simulink model "Two_Zone_MVDC_PSolver"  (R2025b)
settings: Solver=FixedStepDiscrete  StartTime=0.0  StopTime=30  FixedStep=TsELEC  RelTol=1e-3  EnableMultiTasking=on
InitFcn:
  | TsELEC = 25e-6;
  | Ts = 25e-6;
undefined symbols (not defined in the file or in its folder): DiscIntNeverNeededParam, ee_sli_rtmsupport, GABDA, GABDB, GBBDA, GBBDB, gcbh, GPPMA, GPPMB, GPPMC, SADA, SADB, SADC, SADD, SBDA, SBDB, SBDC, SCDA, SCDB, SCDC, SCDD, SDDA, SDDB, SDDC, SDDD, SDDE, TsCont
libraries: fl_lib x97, nesl_utility x73, ee_lib x48, simulink x3, slpidlib x3, eeSmAC1C x2, eePowerMeasurement x2, mcbeeMathTransformLib x2, eeTransforms x1
(part 2 of 4)

== system Two_Zone_MVDC_PSolver/SCDC ==
  SADA : ee_lib/Switches & Breakers/DPST Switch  R_closed=1e-4 Ohm  G_open=1e-6 S  Threshold=0.5 V  Width=0 V  model_dynamics=0  t_on=1e-3 s  t_off=1e-3 s  initial_vT=0 V
      settings: InternalSimscapePortConfiguration="{\"Bottom\":[],\"Left\":[{\"id\":\"vT\",\"label\":\"vT\",\"type\":\"input\"},{\"id\":\"p1\",\"label\":\"\",\"type\":\"foundation.electrical.electrical\"},{\"id\":\"p2\",\"label\":\"\",\"type\":\"foundation.electrical.electrical\"}],\"Right\":[{\"id\":\"n1\",\"label\":\"\",\"type\":\"foundation.electrical.electrical\"},{\"id\":\"n2\",\"label\":\"\",\"type\":\"foundation.electrical.electrical\"}],\"Top\":[]}"
  Simulink-PS Converter : nesl_utility/Simulink-PS Converter  PhysicalDomain=network_engine_domain  SubClassName=ps_input  LeftPortType=input  RightPortType=output  PseudoPeriodic=off  Frequencies=[]  NoiseDistribution=none  NoiseParameters=[]  Unit=1  AffineConversion=off  FilteringAndDerivatives=provide  SimscapeFilterOrder=1  InputFilterTimeConstant=0.001  UdotUserProvided=0
  "+ " : PMIOPort  Side=Right
  + : PMIOPort  Port=2  Side=Left
  "- " : PMIOPort  Port=3  Side=Right
  - : PMIOPort  Port=4  Side=Left
  wires:
  [SCDC] -> Simulink-PS Converter/1
  connections:
  SADA/LConn2 -- +/RConn1
  Simulink-PS Converter/RConn1 -- SADA/LConn1
  SADA/RConn2 -- "- "/RConn1
  SADA/LConn3 -- -/RConn1
  SADA/RConn1 -- "+ "/RConn1

== system Two_Zone_MVDC_PSolver/SCDD ==
  SADA : ee_lib/Switches & Breakers/DPST Switch  R_closed=1e-4 Ohm  G_open=1e-6 S  Threshold=0.5 V  Width=0 V  model_dynamics=0  t_on=1e-3 s  t_off=1e-3 s  initial_vT=0 V
      settings: InternalSimscapePortConfiguration="{\"Bottom\":[],\"Left\":[{\"id\":\"vT\",\"label\":\"vT\",\"type\":\"input\"},{\"id\":\"p1\",\"label\":\"\",\"type\":\"foundation.electrical.electrical\"},{\"id\":\"p2\",\"label\":\"\",\"type\":\"foundation.electrical.electrical\"}],\"Right\":[{\"id\":\"n1\",\"label\":\"\",\"type\":\"foundation.electrical.electrical\"},{\"id\":\"n2\",\"label\":\"\",\"type\":\"foundation.electrical.electrical\"}],\"Top\":[]}"
  Simulink-PS Converter : nesl_utility/Simulink-PS Converter  PhysicalDomain=network_engine_domain  SubClassName=ps_input  LeftPortType=input  RightPortType=output  PseudoPeriodic=off  Frequencies=[]  NoiseDistribution=none  NoiseParameters=[]  Unit=1  AffineConversion=off  FilteringAndDerivatives=provide  SimscapeFilterOrder=1  InputFilterTimeConstant=0.001  UdotUserProvided=0
  "+ " : PMIOPort  Side=Right
  + : PMIOPort  Port=2  Side=Left
  "- " : PMIOPort  Port=3  Side=Right
  - : PMIOPort  Port=4  Side=Left
  wires:
  [SCDD] -> Simulink-PS Converter/1
  connections:
  SADA/RConn1 -- "+ "/RConn1
  SADA/LConn3 -- -/RConn1
  SADA/RConn2 -- "- "/RConn1
  Simulink-PS Converter/RConn1 -- SADA/LConn1
  SADA/LConn2 -- +/RConn1

== system Two_Zone_MVDC_PSolver/SDDA ==
  SDDA : ee_lib/Switches & Breakers/DPST Switch  R_closed=1e-4 Ohm  G_open=1e-6 S  Threshold=0.5 V  Width=0 V  model_dynamics=0  t_on=1e-3 s  t_off=1e-3 s  initial_vT=0 V
      settings: InternalSimscapePortConfiguration="{\"Bottom\":[],\"Left\":[{\"id\":\"vT\",\"label\":\"vT\",\"type\":\"input\"},{\"id\":\"p1\",\"label\":\"\",\"type\":\"foundation.electrical.electrical\"},{\"id\":\"p2\",\"label\":\"\",\"type\":\"foundation.electrical.electrical\"}],\"Right\":[{\"id\":\"n1\",\"label\":\"\",\"type\":\"foundation.electrical.electrical\"},{\"id\":\"n2\",\"label\":\"\",\"type\":\"foundation.electrical.electrical\"}],\"Top\":[]}"
  Simulink-PS Converter : nesl_utility/Simulink-PS Converter  PhysicalDomain=network_engine_domain  SubClassName=ps_input  LeftPortType=input  RightPortType=output  PseudoPeriodic=off  Frequencies=[]  NoiseDistribution=none  NoiseParameters=[]  Unit=1  AffineConversion=off  FilteringAndDerivatives=provide  SimscapeFilterOrder=1  InputFilterTimeConstant=0.001  UdotUserProvided=0
  "+ " : PMIOPort  Side=Right
  + : PMIOPort  Port=2  Side=Left
  "- " : PMIOPort  Port=3  Side=Right
  - : PMIOPort  Port=4  Side=Left
  wires:
  [SDDA] -> Simulink-PS Converter/1
  connections:
  SDDA/LConn2 -- +/RConn1
  Simulink-PS Converter/RConn1 -- SDDA/LConn1
  SDDA/RConn2 -- "- "/RConn1
  SDDA/LConn3 -- -/RConn1
  SDDA/RConn1 -- "+ "/RConn1

== system Two_Zone_MVDC_PSolver/SDDB ==
  SDDB : ee_lib/Switches & Breakers/DPST Switch  R_closed=1e-4 Ohm  G_open=1e-6 S  Threshold=0.5 V  Width=0 V  model_dynamics=0  t_on=1e-3 s  t_off=1e-3 s  initial_vT=0 V
      settings: InternalSimscapePortConfiguration="{\"Bottom\":[],\"Left\":[{\"id\":\"vT\",\"label\":\"vT\",\"type\":\"input\"},{\"id\":\"p1\",\"label\":\"\",\"type\":\"foundation.electrical.electrical\"},{\"id\":\"p2\",\"label\":\"\",\"type\":\"foundation.electrical.electrical\"}],\"Right\":[{\"id\":\"n1\",\"label\":\"\",\"type\":\"foundation.electrical.electrical\"},{\"id\":\"n2\",\"label\":\"\",\"type\":\"foundation.electrical.electrical\"}],\"Top\":[]}"
  Simulink-PS Converter : nesl_utility/Simulink-PS Converter  PhysicalDomain=network_engine_domain  SubClassName=ps_input  LeftPortType=input  RightPortType=output  PseudoPeriodic=off  Frequencies=[]  NoiseDistribution=none  NoiseParameters=[]  Unit=1  AffineConversion=off  FilteringAndDerivatives=provide  SimscapeFilterOrder=1  InputFilterTimeConstant=0.001  UdotUserProvided=0
  "+ " : PMIOPort  Side=Right
  + : PMIOPort  Port=2  Side=Left
  "- " : PMIOPort  Port=3  Side=Right
  - : PMIOPort  Port=4  Side=Left
  wires:
  [SDDB] -> Simulink-PS Converter/1
  connections:
  SDDB/RConn1 -- "+ "/RConn1
  SDDB/LConn3 -- -/RConn1
  SDDB/RConn2 -- "- "/RConn1
  Simulink-PS Converter/RConn1 -- SDDB/LConn1
  SDDB/LConn2 -- +/RConn1

== system Two_Zone_MVDC_PSolver/SDDC ==
  SDDC : ee_lib/Switches & Breakers/DPST Switch  R_closed=1e-4 Ohm  G_open=1e-6 S  Threshold=0.5 V  Width=0 V  model_dynamics=0  t_on=1e-3 s  t_off=1e-3 s  initial_vT=0 V
      settings: InternalSimscapePortConfiguration="{\"Bottom\":[],\"Left\":[{\"id\":\"vT\",\"label\":\"vT\",\"type\":\"input\"},{\"id\":\"p1\",\"label\":\"\",\"type\":\"foundation.electrical.electrical\"},{\"id\":\"p2\",\"label\":\"\",\"type\":\"foundation.electrical.electrical\"}],\"Right\":[{\"id\":\"n1\",\"label\":\"\",\"type\":\"foundation.electrical.electrical\"},{\"id\":\"n2\",\"label\":\"\",\"type\":\"foundation.electrical.electrical\"}],\"Top\":[]}"
  Simulink-PS Converter : nesl_utility/Simulink-PS Converter  PhysicalDomain=network_engine_domain  SubClassName=ps_input  LeftPortType=input  RightPortType=output  PseudoPeriodic=off  Frequencies=[]  NoiseDistribution=none  NoiseParameters=[]  Unit=1  AffineConversion=off  FilteringAndDerivatives=provide  SimscapeFilterOrder=1  InputFilterTimeConstant=0.001  UdotUserProvided=0
  "+ " : PMIOPort  Side=Right
  + : PMIOPort  Port=2  Side=Left
  "- " : PMIOPort  Port=3  Side=Right
  - : PMIOPort  Port=4  Side=Left
  wires:
  [SDDC] -> Simulink-PS Converter/1
  connections:
  SDDC/LConn2 -- +/RConn1
  Simulink-PS Converter/RConn1 -- SDDC/LConn1
  SDDC/RConn2 -- "- "/RConn1
  SDDC/LConn3 -- -/RConn1
  SDDC/RConn1 -- "+ "/RConn1

== system Two_Zone_MVDC_PSolver/SDDD ==
  SDDD : ee_lib/Switches & Breakers/DPST Switch  R_closed=1e-4 Ohm  G_open=1e-6 S  Threshold=0.5 V  Width=0 V  model_dynamics=0  t_on=1e-3 s  t_off=1e-3 s  initial_vT=0 V
      settings: InternalSimscapePortConfiguration="{\"Bottom\":[],\"Left\":[{\"id\":\"vT\",\"label\":\"vT\",\"type\":\"input\"},{\"id\":\"p1\",\"label\":\"\",\"type\":\"foundation.electrical.electrical\"},{\"id\":\"p2\",\"label\":\"\",\"type\":\"foundation.electrical.electrical\"}],\"Right\":[{\"id\":\"n1\",\"label\":\"\",\"type\":\"foundation.electrical.electrical\"},{\"id\":\"n2\",\"label\":\"\",\"type\":\"foundation.electrical.electrical\"}],\"Top\":[]}"
  Simulink-PS Converter : nesl_utility/Simulink-PS Converter  PhysicalDomain=network_engine_domain  SubClassName=ps_input  LeftPortType=input  RightPortType=output  PseudoPeriodic=off  Frequencies=[]  NoiseDistribution=none  NoiseParameters=[]  Unit=1  AffineConversion=off  FilteringAndDerivatives=provide  SimscapeFilterOrder=1  InputFilterTimeConstant=0.001  UdotUserProvided=0
  "+ " : PMIOPort  Side=Right
  + : PMIOPort  Port=2  Side=Left
  "- " : PMIOPort  Port=3  Side=Right
  - : PMIOPort  Port=4  Side=Left
  wires:
  [SDDD] -> Simulink-PS Converter/1
  connections:
  SDDD/RConn1 -- "+ "/RConn1
  SDDD/LConn3 -- -/RConn1
  SDDD/RConn2 -- "- "/RConn1
  Simulink-PS Converter/RConn1 -- SDDD/LConn1
  SDDD/LConn2 -- +/RConn1

== system Two_Zone_MVDC_PSolver/SDDE ==
  SDDE : ee_lib/Switches & Breakers/DPST Switch  R_closed=1e-4 Ohm  G_open=1e-6 S  Threshold=0.5 V  Width=0 V  model_dynamics=0  t_on=1e-3 s  t_off=1e-3 s  initial_vT=0 V
      settings: InternalSimscapePortConfiguration="{\"Bottom\":[],\"Left\":[{\"id\":\"vT\",\"label\":\"vT\",\"type\":\"input\"},{\"id\":\"p1\",\"label\":\"\",\"type\":\"foundation.electrical.electrical\"},{\"id\":\"p2\",\"label\":\"\",\"type\":\"foundation.electrical.electrical\"}],\"Right\":[{\"id\":\"n1\",\"label\":\"\",\"type\":\"foundation.electrical.electrical\"},{\"id\":\"n2\",\"label\":\"\",\"type\":\"foundation.electrical.electrical\"}],\"Top\":[]}"
  Simulink-PS Converter : nesl_utility/Simulink-PS Converter  PhysicalDomain=network_engine_domain  SubClassName=ps_input  LeftPortType=input  RightPortType=output  PseudoPeriodic=off  Frequencies=[]  NoiseDistribution=none  NoiseParameters=[]  Unit=1  AffineConversion=off  FilteringAndDerivatives=provide  SimscapeFilterOrder=1  InputFilterTimeConstant=0.001  UdotUserProvided=0
  "+ " : PMIOPort  Side=Right
  + : PMIOPort  Port=2  Side=Left
  "- " : PMIOPort  Port=3  Side=Right
  - : PMIOPort  Port=4  Side=Left
  wires:
  [SDDE] -> Simulink-PS Converter/1
  connections:
  SDDE/RConn1 -- "+ "/RConn1
  SDDE/LConn3 -- -/RConn1
  SDDE/RConn2 -- "- "/RConn1
  Simulink-PS Converter/RConn1 -- SDDE/LConn1
  SDDE/LConn2 -- +/RConn1

== system Two_Zone_MVDC_PSolver/Subsystem1 ==
  Inductor1 : fl_lib/Electrical/Electrical Elements/Inductor  l=5.32e-6 H  r=0.32e-3 Ohm  g=0 1/Ohm  i_specify=off  i_priority=None  i=0 A  i_nominal_specify=off  i_nominal_value=1  i_nominal_unit=A  v_specify=off  v_priority=None  v=0 V  v_nominal_specify=off  v_nominal_value=1  v_nominal_unit=V  i_L_specify=off  i_L_priority=High  i_L=0 A  i_L_nominal_specify=off  i_L_nominal_value=1  i_L_nominal_unit=A
  Inductor2 : fl_lib/Electrical/Electrical Elements/Inductor  l=5.32e-6 H  r=0.32e-3 Ohm  g=0 1/Ohm  i_specify=off  i_priority=None  i=0 A  i_nominal_specify=off  i_nominal_value=1  i_nominal_unit=A  v_specify=off  v_priority=None  v=0 V  v_nominal_specify=off  v_nominal_value=1  v_nominal_unit=V  i_L_specify=off  i_L_priority=High  i_L=0 A  i_L_nominal_specify=off  i_L_nominal_value=1  i_L_nominal_unit=A
  "+ " : PMIOPort  Side=Left
  + : PMIOPort  Port=2  Side=Right
  - : PMIOPort  Port=3  Side=Left
  "- " : PMIOPort  Port=4  Side=Right
  connections:
  Inductor1/LConn1 -- -/RConn1
  Inductor2/LConn1 -- "+ "/RConn1
  Inductor2/RConn1 -- +/RConn1
  Inductor1/RConn1 -- "- "/RConn1

== system Two_Zone_MVDC_PSolver/Subsystem10 ==
  Current Sensor : fl_lib/Electrical/Electrical Sensors/Current Sensor
  Inductor1 : fl_lib/Electrical/Electrical Elements/Inductor  l=3.47e-6 H  r=0.21e-3 Ohm  g=0 1/Ohm  i_specify=off  i_priority=None  i=0 A  i_nominal_specify=off  i_nominal_value=1  i_nominal_unit=A  v_specify=off  v_priority=None  v=0 V  v_nominal_specify=off  v_nominal_value=1  v_nominal_unit=V  i_L_specify=off  i_L_priority=High  i_L=0 A  i_L_nominal_specify=off  i_L_nominal_value=1  i_L_nominal_unit=A
  Inductor3 : fl_lib/Electrical/Electrical Elements/Inductor  l=3.47e-6 H  r=0.21e-3 Ohm  g=0 1/Ohm  i_specify=off  i_priority=None  i=0 A  i_nominal_specify=off  i_nominal_value=1  i_nominal_unit=A  v_specify=off  v_priority=None  v=0 V  v_nominal_specify=off  v_nominal_value=1  v_nominal_unit=V  i_L_specify=off  i_L_priority=High  i_L=0 A  i_L_nominal_specify=off  i_L_nominal_value=1  i_L_nominal_unit=A
  PS-Simulink Converter : nesl_utility/PS-Simulink Converter  PhysicalDomain=network_engine_domain  SubClassName=ps_output  LeftPortType=input  RightPortType=output  PseudoPeriodic=off  Frequencies=[]  VectorFormat=1-D array  Unit=inherit  AffineConversion=off
  PS-Simulink Converter1 : nesl_utility/PS-Simulink Converter  PhysicalDomain=network_engine_domain  SubClassName=ps_output  LeftPortType=input  RightPortType=output  PseudoPeriodic=off  Frequencies=[]  VectorFormat=1-D array  Unit=inherit  AffineConversion=off
  Product : Product
  Terminator : Terminator
  Voltage Sensor : fl_lib/Electrical/Electrical Sensors/Voltage Sensor
  "+ " : PMIOPort  Side=Left
  + : PMIOPort  Port=2  Side=Right
  - : PMIOPort  Port=3  Side=Left
  "- " : PMIOPort  Port=4  Side=Right
  wires:
  Product/1 -> Terminator/1  "P_CS6"
  PS-Simulink Converter/1 -> Product/1
  PS-Simulink Converter1/1 -> Product/2
  connections:
  Inductor1/LConn1 -- -/RConn1
  Inductor3/LConn1 -- "+ "/RConn1
  Inductor3/RConn1 -- Current Sensor/LConn1
  Current Sensor/RConn2 -- Voltage Sensor/LConn1 -- +/RConn1
  Inductor1/RConn1 -- Voltage Sensor/RConn2 -- "- "/RConn1
  Voltage Sensor/RConn1 -- PS-Simulink Converter1/LConn1
  PS-Simulink Converter/LConn1 -- Current Sensor/RConn1

== system Two_Zone_MVDC_PSolver/Subsystem12 ==
  Inductor1 : fl_lib/Electrical/Electrical Elements/Inductor  l=2.63e-6 H  r=0.16e-3 Ohm  g=0 1/Ohm  i_specify=off  i_priority=None  i=0 A  i_nominal_specify=off  i_nominal_value=1  i_nominal_unit=A  v_specify=off  v_priority=None  v=0 V  v_nominal_specify=off  v_nominal_value=1  v_nominal_unit=V  i_L_specify=off  i_L_priority=High  i_L=0 A  i_L_nominal_specify=off  i_L_nominal_value=1  i_L_nominal_unit=A
  Inductor3 : fl_lib/Electrical/Electrical Elements/Inductor  l=2.63e-6 H  r=0.16e-3 Ohm  g=0 1/Ohm  i_specify=off  i_priority=None  i=0 A  i_nominal_specify=off  i_nominal_value=1  i_nominal_unit=A  v_specify=off  v_priority=None  v=0 V  v_nominal_specify=off  v_nominal_value=1  v_nominal_unit=V  i_L_specify=off  i_L_priority=High  i_L=0 A  i_L_nominal_specify=off  i_L_nominal_value=1  i_L_nominal_unit=A
  "+ " : PMIOPort  Side=Left
  + : PMIOPort  Port=2  Side=Right
  - : PMIOPort  Port=3  Side=Left
  "- " : PMIOPort  Port=4  Side=Right
  connections:
  Inductor1/LConn1 -- -/RConn1
  Inductor3/LConn1 -- "+ "/RConn1
  Inductor3/RConn1 -- +/RConn1
  Inductor1/RConn1 -- "- "/RConn1

== system Two_Zone_MVDC_PSolver/Subsystem13 ==
  Current Sensor : fl_lib/Electrical/Electrical Sensors/Current Sensor
  Inductor1 : fl_lib/Electrical/Electrical Elements/Inductor  l=5e-6 H  r=0.2e-3 Ohm  g=0 1/Ohm  i_specify=off  i_priority=None  i=0 A  i_nominal_specify=off  i_nominal_value=1  i_nominal_unit=A  v_specify=off  v_priority=None  v=0 V  v_nominal_specify=off  v_nominal_value=1  v_nominal_unit=V  i_L_specify=off  i_L_priority=High  i_L=0 A  i_L_nominal_specify=off  i_L_nominal_value=1  i_L_nominal_unit=A
  Inductor3 : fl_lib/Electrical/Electrical Elements/Inductor  l=5e-6 H  r=0.2e-3 Ohm  g=0 1/Ohm  i_specify=off  i_priority=None  i=0 A  i_nominal_specify=off  i_nominal_value=1  i_nominal_unit=A  v_specify=off  v_priority=None  v=0 V  v_nominal_specify=off  v_nominal_value=1  v_nominal_unit=V  i_L_specify=off  i_L_priority=High  i_L=0 A  i_L_nominal_specify=off  i_L_nominal_value=1  i_L_nominal_unit=A
  PS-Simulink Converter : nesl_utility/PS-Simulink Converter  PhysicalDomain=network_engine_domain  SubClassName=ps_output  LeftPortType=input  RightPortType=output  PseudoPeriodic=off  Frequencies=[]  VectorFormat=1-D array  Unit=inherit  AffineConversion=off
  PS-Simulink Converter1 : nesl_utility/PS-Simulink Converter  PhysicalDomain=network_engine_domain  SubClassName=ps_output  LeftPortType=input  RightPortType=output  PseudoPeriodic=off  Frequencies=[]  VectorFormat=1-D array  Unit=inherit  AffineConversion=off
  Product : Product
  Terminator : Terminator
  Voltage Sensor : fl_lib/Electrical/Electrical Sensors/Voltage Sensor
  "+ " : PMIOPort  Side=Left
  + : PMIOPort  Port=2  Side=Right
  - : PMIOPort  Port=3  Side=Left
  "- " : PMIOPort  Port=4  Side=Right
  wires:
  Product/1 -> Terminator/1  "P_CS4"
  PS-Simulink Converter/1 -> Product/1
  PS-Simulink Converter1/1 -> Product/2
  connections:
  Inductor3/LConn1 -- "+ "/RConn1
  Inductor1/LConn1 -- -/RConn1
  Current Sensor/LConn1 -- Inductor3/RConn1
  Current Sensor/RConn2 -- Voltage Sensor/LConn1 -- +/RConn1
  Inductor1/RConn1 -- Voltage Sensor/RConn2 -- "- "/RConn1
  Current Sensor/RConn1 -- PS-Simulink Converter/LConn1
  PS-Simulink Converter1/LConn1 -- Voltage Sensor/RConn1

== system Two_Zone_MVDC_PSolver/Subsystem14 ==
  Inductor1 : fl_lib/Electrical/Electrical Elements/Inductor  l=5.32e-6 H  r=0.32e-3 Ohm  g=0 1/Ohm  i_specify=off  i_priority=None  i=0 A  i_nominal_specify=off  i_nominal_value=1  i_nominal_unit=A  v_specify=off  v_priority=None  v=0 V  v_nominal_specify=off  v_nominal_value=1  v_nominal_unit=V  i_L_specify=off  i_L_priority=High  i_L=0 A  i_L_nominal_specify=off  i_L_nominal_value=1  i_L_nominal_unit=A
  Inductor2 : fl_lib/Electrical/Electrical Elements/Inductor  l=5.32e-6 H  r=0.32e-3 Ohm  g=0 1/Ohm  i_specify=off  i_priority=None  i=0 A  i_nominal_specify=off  i_nominal_value=1  i_nominal_unit=A  v_specify=off  v_priority=None  v=0 V  v_nominal_specify=off  v_nominal_value=1  v_nominal_unit=V  i_L_specify=off  i_L_priority=High  i_L=0 A  i_L_nominal_specify=off  i_L_nominal_value=1  i_L_nominal_unit=A
  "+ " : PMIOPort  Side=Left
  + : PMIOPort  Port=2  Side=Right
  - : PMIOPort  Port=3  Side=Left
  "- " : PMIOPort  Port=4  Side=Right
  connections:
  Inductor1/LConn1 -- -/RConn1
  Inductor2/LConn1 -- "+ "/RConn1
  Inductor2/RConn1 -- +/RConn1
  Inductor1/RConn1 -- "- "/RConn1

== system Two_Zone_MVDC_PSolver/Subsystem15 ==
  Inductor1 : fl_lib/Electrical/Electrical Elements/Inductor  l=5.32e-6 H  r=0.32e-3 Ohm  g=0 1/Ohm  i_specify=off  i_priority=None  i=0 A  i_nominal_specify=off  i_nominal_value=1  i_nominal_unit=A  v_specify=off  v_priority=None  v=0 V  v_nominal_specify=off  v_nominal_value=1  v_nominal_unit=V  i_L_specify=off  i_L_priority=High  i_L=0 A  i_L_nominal_specify=off  i_L_nominal_value=1  i_L_nominal_unit=A
  Inductor2 : fl_lib/Electrical/Electrical Elements/Inductor  l=5.32e-6 H  r=0.32e-3 Ohm  g=0 1/Ohm  i_specify=off  i_priority=None  i=0 A  i_nominal_specify=off  i_nominal_value=1  i_nominal_unit=A  v_specify=off  v_priority=None  v=0 V  v_nominal_specify=off  v_nominal_value=1  v_nominal_unit=V  i_L_specify=off  i_L_priority=High  i_L=0 A  i_L_nominal_specify=off  i_L_nominal_value=1  i_L_nominal_unit=A
  "+ " : PMIOPort  Side=Left
  + : PMIOPort  Port=2  Side=Right
  - : PMIOPort  Port=3  Side=Left
  "- " : PMIOPort  Port=4  Side=Right
  connections:
  Inductor1/RConn1 -- "- "/RConn1
  Inductor2/RConn1 -- +/RConn1
  Inductor2/LConn1 -- "+ "/RConn1
  Inductor1/LConn1 -- -/RConn1

== system Two_Zone_MVDC_PSolver/Subsystem16 ==
  Inductor1 : fl_lib/Electrical/Electrical Elements/Inductor  l=5.32e-6 H  r=0.32e-3 Ohm  g=0 1/Ohm  i_specify=off  i_priority=None  i=0 A  i_nominal_specify=off  i_nominal_value=1  i_nominal_unit=A  v_specify=off  v_priority=None  v=0 V  v_nominal_specify=off  v_nominal_value=1  v_nominal_unit=V  i_L_specify=off  i_L_priority=High  i_L=0 A  i_L_nominal_specify=off  i_L_nominal_value=1  i_L_nominal_unit=A
  Inductor2 : fl_lib/Electrical/Electrical Elements/Inductor  l=5.32e-6 H  r=0.32e-3 Ohm  g=0 1/Ohm  i_specify=off  i_priority=None  i=0 A  i_nominal_specify=off  i_nominal_value=1  i_nominal_unit=A  v_specify=off  v_priority=None  v=0 V  v_nominal_specify=off  v_nominal_value=1  v_nominal_unit=V  i_L_specify=off  i_L_priority=High  i_L=0 A  i_L_nominal_specify=off  i_L_nominal_value=1  i_L_nominal_unit=A
  "+ " : PMIOPort  Side=Left
  + : PMIOPort  Port=2  Side=Right
  - : PMIOPort  Port=3  Side=Left
  "- " : PMIOPort  Port=4  Side=Right
  connections:
  Inductor1/LConn1 -- -/RConn1
  Inductor2/LConn1 -- "+ "/RConn1
  Inductor2/RConn1 -- +/RConn1
  Inductor1/RConn1 -- "- "/RConn1

== system Two_Zone_MVDC_PSolver/Subsystem2 ==
  Current Sensor : fl_lib/Electrical/Electrical Sensors/Current Sensor
  Inductor1 : fl_lib/Electrical/Electrical Elements/Inductor  l=5e-6 H  r=0.2e-3 Ohm  g=0 1/Ohm  i_specify=off  i_priority=None  i=0 A  i_nominal_specify=off  i_nominal_value=1  i_nominal_unit=A  v_specify=off  v_priority=None  v=0 V  v_nominal_specify=off  v_nominal_value=1  v_nominal_unit=V  i_L_specify=off  i_L_priority=High  i_L=0 A  i_L_nominal_specify=off  i_L_nominal_value=1  i_L_nominal_unit=A
  Inductor3 : fl_lib/Electrical/Electrical Elements/Inductor  l=5e-6 H  r=0.2e-3 Ohm  g=0 1/Ohm  i_specify=off  i_priority=None  i=0 A  i_nominal_specify=off  i_nominal_value=1  i_nominal_unit=A  v_specify=off  v_priority=None  v=0 V  v_nominal_specify=off  v_nominal_value=1  v_nominal_unit=V  i_L_specify=off  i_L_priority=High  i_L=0 A  i_L_nominal_specify=off  i_L_nominal_value=1  i_L_nominal_unit=A
  PS-Simulink Converter : nesl_utility/PS-Simulink Converter  PhysicalDomain=network_engine_domain  SubClassName=ps_output  LeftPortType=input  RightPortType=output  PseudoPeriodic=off  Frequencies=[]  VectorFormat=1-D array  Unit=inherit  AffineConversion=off
  PS-Simulink Converter1 : nesl_utility/PS-Simulink Converter  PhysicalDomain=network_engine_domain  SubClassName=ps_output  LeftPortType=input  RightPortType=output  PseudoPeriodic=off  Frequencies=[]  VectorFormat=1-D array  Unit=inherit  AffineConversion=off
  Product : Product
  Terminator : Terminator
  Voltage Sensor : fl_lib/Electrical/Electrical Sensors/Voltage Sensor
  "+ " : PMIOPort  Side=Left
  + : PMIOPort  Port=2  Side=Right
  - : PMIOPort  Port=3  Side=Left
  "- " : PMIOPort  Port=4  Side=Right
  wires:
  Product/1 -> Terminator/1  "P_CS8"
  PS-Simulink Converter/1 -> Product/1
  PS-Simulink Converter1/1 -> Product/2
  connections:
  Inductor1/LConn1 -- -/RConn1
  Inductor3/LConn1 -- "+ "/RConn1
  Current Sensor/LConn1 -- Inductor3/RConn1
  Current Sensor/RConn2 -- Voltage Sensor/LConn1 -- +/RConn1
  Inductor1/RConn1 -- Voltage Sensor/RConn2 -- "- "/RConn1
  Voltage Sensor/RConn1 -- PS-Simulink Converter1/LConn1
  Current Sensor/RConn1 -- PS-Simulink Converter/LConn1

== system Two_Zone_MVDC_PSolver/Subsystem5 ==
  Inductor1 : fl_lib/Electrical/Electrical Elements/Inductor  l=5.32e-6 H  r=0.32e-3 Ohm  g=0 1/Ohm  i_specify=off  i_priority=None  i=0 A  i_nominal_specify=off  i_nominal_value=1  i_nominal_unit=A  v_specify=off  v_priority=None  v=0 V  v_nominal_specify=off  v_nominal_value=1  v_nominal_unit=V  i_L_specify=off  i_L_priority=High  i_L=0 A  i_L_nominal_specify=off  i_L_nominal_value=1  i_L_nominal_unit=A
  Inductor2 : fl_lib/Electrical/Electrical Elements/Inductor  l=5.32e-6 H  r=0.32e-3 Ohm  g=0 1/Ohm  i_specify=off  i_priority=None  i=0 A  i_nominal_specify=off  i_nominal_value=1  i_nominal_unit=A  v_specify=off  v_priority=None  v=0 V  v_nominal_specify=off  v_nominal_value=1  v_nominal_unit=V  i_L_specify=off  i_L_priority=High  i_L=0 A  i_L_nominal_specify=off  i_L_nominal_value=1  i_L_nominal_unit=A
  "+ " : PMIOPort  Side=Left
  + : PMIOPort  Port=2  Side=Right
  - : PMIOPort  Port=3  Side=Left
  "- " : PMIOPort  Port=4  Side=Right
  connections:
  Inductor1/RConn1 -- "- "/RConn1
  Inductor2/RConn1 -- +/RConn1
  Inductor2/LConn1 -- "+ "/RConn1
  Inductor1/LConn1 -- -/RConn1

== system Two_Zone_MVDC_PSolver/Subsystem6 ==
  Inductor1 : fl_lib/Electrical/Electrical Elements/Inductor  l=2.63e-6 H  r=0.16e-3 Ohm  g=0 1/Ohm  i_specify=off  i_priority=None  i=0 A  i_nominal_specify=off  i_nominal_value=1  i_nominal_unit=A  v_specify=off  v_priority=None  v=0 V  v_nominal_specify=off  v_nominal_value=1  v_nominal_unit=V  i_L_specify=off  i_L_priority=High  i_L=0 A  i_L_nominal_specify=off  i_L_nominal_value=1  i_L_nominal_unit=A
  Inductor3 : fl_lib/Electrical/Electrical Elements/Inductor  l=2.63e-6 H  r=0.16e-3 Ohm  g=0 1/Ohm  i_specify=off  i_priority=None  i=0 A  i_nominal_specify=off  i_nominal_value=1  i_nominal_unit=A  v_specify=off  v_priority=None  v=0 V  v_nominal_specify=off  v_nominal_value=1  v_nominal_unit=V  i_L_specify=off  i_L_priority=High  i_L=0 A  i_L_nominal_specify=off  i_L_nominal_value=1  i_L_nominal_unit=A
  "+ " : PMIOPort  Side=Left
  + : PMIOPort  Port=2  Side=Right
  - : PMIOPort  Port=3  Side=Left
  "- " : PMIOPort  Port=4  Side=Right
  connections:
  Inductor1/LConn1 -- -/RConn1
  Inductor3/LConn1 -- "+ "/RConn1
  Inductor3/RConn1 -- +/RConn1
  Inductor1/RConn1 -- "- "/RConn1

== system Two_Zone_MVDC_PSolver/Subsystem8 ==
  Inductor1 : fl_lib/Electrical/Electrical Elements/Inductor  l=2.63e-6 H  r=0.16e-3 Ohm  g=0 1/Ohm  i_specify=off  i_priority=None  i=0 A  i_nominal_specify=off  i_nominal_value=1  i_nominal_unit=A  v_specify=off  v_priority=None  v=0 V  v_nominal_specify=off  v_nominal_value=1  v_nominal_unit=V  i_L_specify=off  i_L_priority=High  i_L=0 A  i_L_nominal_specify=off  i_L_nominal_value=1  i_L_nominal_unit=A
  Inductor3 : fl_lib/Electrical/Electrical Elements/Inductor  l=2.63e-6 H  r=0.16e-3 Ohm  g=0 1/Ohm  i_specify=off  i_priority=None  i=0 A  i_nominal_specify=off  i_nominal_value=1  i_nominal_unit=A  v_specify=off  v_priority=None  v=0 V  v_nominal_specify=off  v_nominal_value=1  v_nominal_unit=V  i_L_specify=off  i_L_priority=High  i_L=0 A  i_L_nominal_specify=off  i_L_nominal_value=1  i_L_nominal_unit=A
  "+ " : PMIOPort  Side=Left
  + : PMIOPort  Port=2  Side=Right
  - : PMIOPort  Port=3  Side=Left
  "- " : PMIOPort  Port=4  Side=Right
  connections:
  Inductor1/RConn1 -- "- "/RConn1
  Inductor3/RConn1 -- +/RConn1
  Inductor3/LConn1 -- "+ "/RConn1
  Inductor1/LConn1 -- -/RConn1

== system Two_Zone_MVDC_PSolver/Subsystem9 ==
  Current Sensor : fl_lib/Electrical/Electrical Sensors/Current Sensor
  Inductor1 : fl_lib/Electrical/Electrical Elements/Inductor  l=3.47e-6 H  r=0.21e-3 Ohm  g=0 1/Ohm  i_specify=off  i_priority=None  i=0 A  i_nominal_specify=off  i_nominal_value=1  i_nominal_unit=A  v_specify=off  v_priority=None  v=0 V  v_nominal_specify=off  v_nominal_value=1  v_nominal_unit=V  i_L_specify=off  i_L_priority=High  i_L=0 A  i_L_nominal_specify=off  i_L_nominal_value=1  i_L_nominal_unit=A
  Inductor3 : fl_lib/Electrical/Electrical Elements/Inductor  l=3.47e-6 H  r=0.21e-3 Ohm  g=0 1/Ohm  i_specify=off  i_priority=None  i=0 A  i_nominal_specify=off  i_nominal_value=1  i_nominal_unit=A  v_specify=off  v_priority=None  v=0 V  v_nominal_specify=off  v_nominal_value=1  v_nominal_unit=V  i_L_specify=off  i_L_priority=High  i_L=0 A  i_L_nominal_specify=off  i_L_nominal_value=1  i_L_nominal_unit=A
  PS-Simulink Converter : nesl_utility/PS-Simulink Converter  PhysicalDomain=network_engine_domain  SubClassName=ps_output  LeftPortType=input  RightPortType=output  PseudoPeriodic=off  Frequencies=[]  VectorFormat=1-D array  Unit=inherit  AffineConversion=off
  PS-Simulink Converter1 : nesl_utility/PS-Simulink Converter  PhysicalDomain=network_engine_domain  SubClassName=ps_output  LeftPortType=input  RightPortType=output  PseudoPeriodic=off  Frequencies=[]  VectorFormat=1-D array  Unit=inherit  AffineConversion=off
  Product : Product
  Terminator : Terminator
  Voltage Sensor : fl_lib/Electrical/Electrical Sensors/Voltage Sensor
  "+ " : PMIOPort  Side=Left
  + : PMIOPort  Port=2  Side=Right
  - : PMIOPort  Port=3  Side=Left
  "- " : PMIOPort  Port=4  Side=Right
  wires:
  PS-Simulink Converter/1 -> Product/1
  PS-Simulink Converter1/1 -> Product/2
  Product/1 -> Terminator/1  "P_CS2"
  connections:
  Inductor3/LConn1 -- "+ "/RConn1
  Inductor1/LConn1 -- -/RConn1
  Inductor1/RConn1 -- Voltage Sensor/RConn2 -- "- "/RConn1
  Current Sensor/LConn1 -- Inductor3/RConn1
  Current Sensor/RConn2 -- Voltage Sensor/LConn1 -- +/RConn1
  PS-Simulink Converter/LConn1 -- Current Sensor/RConn1
  PS-Simulink Converter1/LConn1 -- Voltage Sensor/RConn1

== system Two_Zone_MVDC_PSolver/PGM1/Gas turbine ==
  " AC1C" : Subsystem
  GAST : Subsystem
  Inertia : ee_lib/Electromechanical/Mechanical/Machine Inertia  SRated=36e6 V*A  FRated=60 Hz  nPolePairs=1  inertia_option=2  J=27548 kg*m^2  H=4 s*W/V/A  damper_option=2  D=39.0509 N*m/(rad/s)  pu_D=0.01  initialization_option=2  fMechanical0=60 Hz  fElectrical0=60 Hz
      settings: LogSimulationData=on  InternalSimscapePortConfiguration="{\"Bottom\":[],\"Left\":[{\"id\":\"R\",\"label\":\"R\",\"type\":\"foundation.mechanical.rotational.rotational\"}],\"Right\":[],\"Top\":[]}"
  Synchronous Machine Salient Pole : ee_lib/Electromechanical/Synchronous/Synchronous Machine Salient Pole  port_option=ee.enum.threePhasePort.composite  SRated=36e6 V*A  VRated=13.8e3 V  FRated=60 Hz  nPolePairs=1  param_option=ee.enum.sm.parameterization.standard  fieldCircuitParameterization_option=ee.enum.sm.fieldparameterization.current  baseEfd=216.54 V  baseIfd=200 A  zero_sequence=ee.enum.park.zerosequence.exclude  axes_param=ee.enum.rotorangle.daxis  Ladu=0.9  Laqu=0.55  L0=0.15  Ll=0.15  Ra=0.006  Lfd=0.2571  Rfd=0.0006  L1d=0.2  R1d=0.0354  L1q=0.2567  R1q=0.0428  Xl=0.08  Xd=1.352  Xq=0.836  X0=0.15  Xdd=0.296  Xddd=0.148  Xqdd=0.122  d_option=ee.enum.circuit.open  Td0d=4.141 s  Tdd=1.75 s  Td0dd=0.027 s  Tddd=0.0214 s  q_option=ee.enum.circuit.open  Tq0dd=0.184 s  Tqdd=0.0232 s  saturation_option=ee.enum.saturation.exclude  saturation_ifd=[0, .48, .76, 1.38, 1.79]  saturation_Vag=[0, .43, .59, .71, .76]  initialization_option=ee.enum.sm.initialization.electrical  source_type=ee.enum.sm.load_flow_source_type.Swing  Vmag0=13.8e3 V  Vang0=0 deg  Pt0=2e6 V*A  Qt0=0 V*A  minimum_pu=0.95  phase_search_range=[-30, 30] deg  gmin=1e-6 S  connection_option=ee.enum.Connection.wye  num_q_dampers=1  rotor_offset=-pi / 2 rad  pu_psid_specify=off  pu_psid_priority=None  pu_psid=0  pu_psid_nominal_specify=off  pu_psid_nominal_value=1  pu_psid_nominal_unit=1  pu_psiq_specify=off  pu_psiq_priority=None  pu_psiq=0  pu_psiq_nominal_specify=off  pu_psiq_nominal_value=1  pu_psiq_nominal_unit=1  pu_psifd_specify=off  pu_psifd_priority=None  pu_psifd=0  pu_psifd_nominal_specify=off  pu_psifd_nominal_value=1  pu_psifd_nominal_unit=1  pu_psi1d_specify=off  pu_psi1d_priority=None  pu_psi1d=0  pu_psi1d_nominal_specify=off  pu_psi1d_nominal_value=1  pu_psi1d_nominal_unit=1  pu_psi1q_specify=off  pu_psi1q_priority=None  pu_psi1q=0  pu_psi1q_nominal_specify=off  pu_psi1q_nominal_value=1  pu_psi1q_nominal_unit=1  angular_position_diff_specify=off  angular_position_diff_priority=None  angular_position_diff=18 deg  angular_position_diff_nominal_specify=off  angular_position_diff_nominal_value=1  angular_position_diff_nominal_unit=deg  Tmeas=298.15 K  alpha=3.93e-3 1/K  stator_thermal_mass=100 J/K  rotor_thermal_mass=200 J/K  temperatureA_specify=off  temperatureA_priority=High  temperatureA=25 degC  temperatureA_nominal_specify=off  temperatureA_nominal_value=1  temperatureA_nominal_unit=degC  temperatureB_specify=off  temperatureB_priority=High  temperatureB=25 degC  temperatureB_nominal_specify=off  temperatureB_nominal_value=1  temperatureB_nominal_unit=degC  temperatureC_specify=off  temperatureC_priority=High  temperatureC=25 degC  temperatureC_nominal_specify=off  temperatureC_nominal_value=1  temperatureC_nominal_unit=degC  temperatureR_specify=off  temperatureR_priority=High  temperatureR=25 degC  temperatureR_nominal_specify=off  temperatureR_nominal_value=1  temperatureR_nominal_unit=degC
      settings: InternalSimscapePortConfiguration="{\"Bottom\":[],\"Left\":[{\"id\":\"fd_p\",\"label\":\"fd+\",\"type\":\"foundation.electrical.electrical\"},{\"id\":\"fd_n\",\"label\":\"fd-\",\"type\":\"foundation.electrical.electrical\"},{\"id\":\"R\",\"label\":\"R\",\"type\":\"foundation.mechanical.rotational.rotational\"},{\"id\":\"C\",\"label\":\"C\",\"type\":\"foundation.mechanical.rotational.rotational\"}],\"Right\":[{\"id\":\"pu_output\",\"label\":\"pu\",\"type\":\"output\"},{\"id\":\"N\",\"label\":\"~\",\"type\":\"foundation.electrical.three_phase\"}],\"Top\":[]}"
  meas : PMIOPort  Side=Left
  ~ : PMIOPort  Port=2  Side=Right
  connections:
  " AC1C"/RConn1 -- Synchronous Machine Salient Pole/LConn1
  " AC1C"/LConn1 -- Synchronous Machine Salient Pole/RConn1 -- meas/RConn1
  " AC1C"/RConn2 -- Synchronous Machine Salient Pole/LConn2
  Synchronous Machine Salient Pole/RConn2 -- ~/RConn1
  Inertia/LConn1 -- GAST/RConn1 -- Synchronous Machine Salient Pole/LConn3
  GAST/RConn2 -- Synchronous Machine Salient Pole/LConn4

== system Two_Zone_MVDC_PSolver/PGM1/Subsystem ==
  Controlled Current Source : fl_lib/Electrical/Electrical Sources/Controlled Current Source
  Controlled Current Source1 : fl_lib/Electrical/Electrical Sources/Controlled Current Source
  Controlled Current Source2 : fl_lib/Electrical/Electrical Sources/Controlled Current Source
  Electrical Reference2 : fl_lib/Electrical/Electrical Elements/Electrical Reference
  Phase Splitter : ee_lib/Connectors & References/Phase Splitter
  Three Element Demux : fl_lib/Physical Signals/Nonlinear Operators/PS Three-Element Demux
      settings: InternalSimscapePortConfiguration="{\"Bottom\":[],\"Left\":[{\"id\":\"abc\",\"label\":\"abc\",\"type\":\"input\"}],\"Right\":[{\"id\":\"a\",\"label\":\"a\",\"type\":\"output\"},{\"id\":\"b\",\"label\":\"b\",\"type\":\"output\"},{\"id\":\"c\",\"label\":\"c\",\"type\":\"output\"}],\"Top\":[]}"
  ~ : PMIOPort  Side=Right
  mod : PMIOPort  Port=2  Side=Left
  connections:
  Three Element Demux/LConn1 -- mod/RConn1
  Three Element Demux/RConn1 -- Controlled Current Source/RConn1
  Three Element Demux/RConn2 -- Controlled Current Source1/RConn1
  Controlled Current Source2/RConn1 -- Three Element Demux/RConn3
  Phase Splitter/RConn3 -- Controlled Current Source2/LConn1
  ~/RConn1 -- Phase Splitter/LConn1
  Phase Splitter/RConn2 -- Controlled Current Source1/LConn1
  Phase Splitter/RConn1 -- Controlled Current Source/LConn1
  Controlled Current Source2/RConn2 -- Controlled Current Source1/RConn2 -- Controlled Current Source/RConn2 -- Electrical Reference2/LConn1

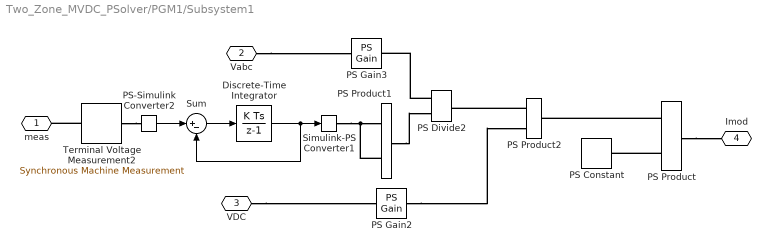
== system Two_Zone_MVDC_PSolver/PGM1/Subsystem1 ==
  Discrete-Time Integrator : DiscreteIntegrator  gainval=200  InitialCondition=1  SampleTime=-1  ICPrevOutput=DiscIntNeverNeededParam  ICPrevScaledInput=DiscIntNeverNeededParam
  PS Constant : fl_lib/Physical Signals/Sources/PS Constant  constant=-12/13.8 1/V/A
  PS Divide2 : fl_lib/Physical Signals/Functions/PS Divide
  PS Gain2 : fl_lib/Physical Signals/Functions/PS Gain  gain=1/12e3 1/V
  PS Gain3 : fl_lib/Physical Signals/Functions/PS Gain  gain=1/13.8e3
  PS Product : fl_lib/Physical Signals/Functions/PS Product
  PS Product1 : fl_lib/Physical Signals/Functions/PS Product
  PS Product2 : fl_lib/Physical Signals/Functions/PS Product
  PS-Simulink Converter2 : nesl_utility/PS-Simulink Converter  PhysicalDomain=network_engine_domain  SubClassName=ps_output  LeftPortType=input  RightPortType=output  PseudoPeriodic=off  Frequencies=[]  VectorFormat=1-D array  Unit=inherit  AffineConversion=off
  Simulink-PS Converter1 : nesl_utility/Simulink-PS Converter  PhysicalDomain=network_engine_domain  SubClassName=ps_input  LeftPortType=input  RightPortType=output  PseudoPeriodic=off  Frequencies=[]  NoiseDistribution=none  NoiseParameters=[]  Unit=1  AffineConversion=off  FilteringAndDerivatives=provide  SimscapeFilterOrder=1  InputFilterTimeConstant=0.001  UdotUserProvided=0
  Sum : Sum  Inputs=|+-
  Terminal Voltage Measurement2 : ee_lib/Electromechanical/Synchronous/Synchronous Machine Measurement  output_idx=14
      settings: LogSimulationData=on  InternalSimscapePortConfiguration="{\"Bottom\":[],\"Left\":[{\"id\":\"pu_input\",\"label\":\"pu\",\"type\":\"input\"}],\"Right\":[{\"id\":\"pu_output\",\"label\":\"o\",\"type\":\"output\"}],\"Top\":[]}"
  meas : PMIOPort  Side=Left
  Vabc : PMIOPort  Port=2  Side=Left
  VDC : PMIOPort  Port=3  Side=Right
  Imod : PMIOPort  Port=4  Side=Right
  wires:
  Sum/1 -> Discrete-Time Integrator/1
  Discrete-Time Integrator/1 -> Sum/2, Simulink-PS Converter1/1
  PS-Simulink Converter2/1 -> Sum/1
  connections:
  PS Product1/RConn1 -- PS Divide2/LConn2
  PS Product/LConn1 -- PS Product2/RConn1
  Vabc/RConn1 -- PS Gain3/LConn1
  PS Gain2/RConn1 -- PS Product2/LConn2
  PS Product/RConn1 -- Imod/RConn1
  VDC/RConn1 -- PS Gain2/LConn1
  PS Product2/LConn1 -- PS Divide2/RConn1
  PS Product/LConn2 -- PS Constant/RConn1
  Terminal Voltage Measurement2/LConn1 -- meas/RConn1
  PS Divide2/LConn1 -- PS Gain3/RConn1
  Terminal Voltage Measurement2/RConn1 -- PS-Simulink Converter2/LConn1
  Simulink-PS Converter1/RConn1 -- PS Product1/LConn2 -- PS Product1/LConn1

== system Two_Zone_MVDC_PSolver/PGM1/breaker status ==
  In1 : Inport
  Demux : Demux  Outputs=[5 4]
  Demux1 : Demux
  Demux2 : Demux  Outputs=5
  tag scope: GABDA=global, GABDB=global, SADA=global, SADB=global, SADC=global, SADD=global, SBDA=global, SBDB=global, SBDC=global
  wires:
  Demux1/4 -> [GABDB]
  Demux1/3 -> [SBDC]
  Demux1/2 -> [SBDB]
  Demux1/1 -> [SBDA]
  Demux/2 -> Demux1/1
  Demux/1 -> Demux2/1
  In1/1 -> Demux/1
  Demux2/4 -> [SADD]
  Demux2/3 -> [SADC]
  Demux2/1 -> [SADA]
  Demux2/2 -> [SADB]
  Demux2/5 -> [GABDA]

== system Two_Zone_MVDC_PSolver/PGM1/breaker status Zone 1 ==
  Constant1 : Constant  Value=SBDA  SampleTime=Ts
  Constant2 : Constant  Value=SADA  SampleTime=Ts
  Constant3 : Constant  Value=SADB  SampleTime=Ts
  Constant4 : Constant  Value=SADC  SampleTime=Ts
  Constant5 : Constant  Value=SADD  SampleTime=Ts
  Constant6 : Constant  Value=GABDA  SampleTime=Ts
  Constant7 : Constant  Value=SBDB  SampleTime=Ts
  Constant8 : Constant  Value=SBDC  SampleTime=Ts
  Constant9 : Constant  Value=GABDB  SampleTime=Ts
  Mux : Mux  Inputs=[5 4]
  Mux1 : Mux  Inputs=5
  Mux2 : Mux
  status : Outport  VectorParamsAs1DForOutWhenUnconnected=off
  wires:
  Constant5/1 -> Mux1/4  "SADD"
  Constant2/1 -> Mux1/1  "SADA"
  Constant3/1 -> Mux1/2  "SADB"
  Constant4/1 -> Mux1/3  "SADC"
  Constant6/1 -> Mux1/5  "GABDA"
  Constant1/1 -> Mux2/1  "SBDA"
  Constant7/1 -> Mux2/2  "SBDB"
  Constant8/1 -> Mux2/3  "SBDC"
  Constant9/1 -> Mux2/4  "GABDB"
  Mux/1 -> status/1
  Mux1/1 -> Mux/1
  Mux2/1 -> Mux/2

== system Two_Zone_MVDC_PSolver/PGM2/Gas turbine ==
  " AC1C" : Subsystem
  GAST : Subsystem
  Inertia : ee_lib/Electromechanical/Mechanical/Machine Inertia  SRated=36e6 V*A  FRated=60 Hz  nPolePairs=1  inertia_option=2  J=27548 kg*m^2  H=4 s*W/V/A  damper_option=2  D=39.0509 N*m/(rad/s)  pu_D=0.01  initialization_option=2  fMechanical0=60 Hz  fElectrical0=60 Hz
      settings: LogSimulationData=on  InternalSimscapePortConfiguration="{\"Bottom\":[],\"Left\":[{\"id\":\"R\",\"label\":\"R\",\"type\":\"foundation.mechanical.rotational.rotational\"}],\"Right\":[],\"Top\":[]}"
  Synchronous Machine Salient Pole : ee_lib/Electromechanical/Synchronous/Synchronous Machine Salient Pole  port_option=ee.enum.threePhasePort.composite  SRated=36e6 V*A  VRated=13.8e3 V  FRated=60 Hz  nPolePairs=1  param_option=ee.enum.sm.parameterization.standard  fieldCircuitParameterization_option=ee.enum.sm.fieldparameterization.current  baseEfd=216.54 V  baseIfd=200 A  zero_sequence=ee.enum.park.zerosequence.exclude  axes_param=ee.enum.rotorangle.daxis  Ladu=0.9  Laqu=0.55  L0=0.15  Ll=0.15  Ra=0.006  Lfd=0.2571  Rfd=0.0006  L1d=0.2  R1d=0.0354  L1q=0.2567  R1q=0.0428  Xl=0.08  Xd=1.352  Xq=0.836  X0=0.15  Xdd=0.296  Xddd=0.148  Xqdd=0.122  d_option=ee.enum.circuit.open  Td0d=4.141 s  Tdd=1.75 s  Td0dd=0.027 s  Tddd=0.0214 s  q_option=ee.enum.circuit.open  Tq0dd=0.184 s  Tqdd=0.0232 s  saturation_option=ee.enum.saturation.exclude  saturation_ifd=[0, .48, .76, 1.38, 1.79]  saturation_Vag=[0, .43, .59, .71, .76]  initialization_option=ee.enum.sm.initialization.electrical  source_type=ee.enum.sm.load_flow_source_type.Swing  Vmag0=13.8e3 V  Vang0=0 deg  Pt0=2e6 V*A  Qt0=0 V*A  minimum_pu=0.95  phase_search_range=[-30, 30] deg  gmin=1e-6 S  connection_option=ee.enum.Connection.wye  num_q_dampers=1  rotor_offset=-pi / 2 rad  pu_psid_specify=off  pu_psid_priority=None  pu_psid=0  pu_psid_nominal_specify=off  pu_psid_nominal_value=1  pu_psid_nominal_unit=1  pu_psiq_specify=off  pu_psiq_priority=None  pu_psiq=0  pu_psiq_nominal_specify=off  pu_psiq_nominal_value=1  pu_psiq_nominal_unit=1  pu_psifd_specify=off  pu_psifd_priority=None  pu_psifd=0  pu_psifd_nominal_specify=off  pu_psifd_nominal_value=1  pu_psifd_nominal_unit=1  pu_psi1d_specify=off  pu_psi1d_priority=None  pu_psi1d=0  pu_psi1d_nominal_specify=off  pu_psi1d_nominal_value=1  pu_psi1d_nominal_unit=1  pu_psi1q_specify=off  pu_psi1q_priority=None  pu_psi1q=0  pu_psi1q_nominal_specify=off  pu_psi1q_nominal_value=1  pu_psi1q_nominal_unit=1  angular_position_diff_specify=off  angular_position_diff_priority=None  angular_position_diff=18 deg  angular_position_diff_nominal_specify=off  angular_position_diff_nominal_value=1  angular_position_diff_nominal_unit=deg  Tmeas=298.15 K  alpha=3.93e-3 1/K  stator_thermal_mass=100 J/K  rotor_thermal_mass=200 J/K  temperatureA_specify=off  temperatureA_priority=High  temperatureA=25 degC  temperatureA_nominal_specify=off  temperatureA_nominal_value=1  temperatureA_nominal_unit=degC  temperatureB_specify=off  temperatureB_priority=High  temperatureB=25 degC  temperatureB_nominal_specify=off  temperatureB_nominal_value=1  temperatureB_nominal_unit=degC  temperatureC_specify=off  temperatureC_priority=High  temperatureC=25 degC  temperatureC_nominal_specify=off  temperatureC_nominal_value=1  temperatureC_nominal_unit=degC  temperatureR_specify=off  temperatureR_priority=High  temperatureR=25 degC  temperatureR_nominal_specify=off  temperatureR_nominal_value=1  temperatureR_nominal_unit=degC
      settings: InternalSimscapePortConfiguration="{\"Bottom\":[],\"Left\":[{\"id\":\"fd_p\",\"label\":\"fd+\",\"type\":\"foundation.electrical.electrical\"},{\"id\":\"fd_n\",\"label\":\"fd-\",\"type\":\"foundation.electrical.electrical\"},{\"id\":\"R\",\"label\":\"R\",\"type\":\"foundation.mechanical.rotational.rotational\"},{\"id\":\"C\",\"label\":\"C\",\"type\":\"foundation.mechanical.rotational.rotational\"}],\"Right\":[{\"id\":\"pu_output\",\"label\":\"pu\",\"type\":\"output\"},{\"id\":\"N\",\"label\":\"~\",\"type\":\"foundation.electrical.three_phase\"}],\"Top\":[]}"
  meas : PMIOPort  Side=Left
  ~ : PMIOPort  Port=2  Side=Right
  connections:
  " AC1C"/RConn1 -- Synchronous Machine Salient Pole/LConn1
  " AC1C"/LConn1 -- Synchronous Machine Salient Pole/RConn1 -- meas/RConn1
  " AC1C"/RConn2 -- Synchronous Machine Salient Pole/LConn2
  Synchronous Machine Salient Pole/RConn2 -- ~/RConn1
  Inertia/LConn1 -- Synchronous Machine Salient Pole/LConn3 -- GAST/RConn1
  GAST/RConn2 -- Synchronous Machine Salient Pole/LConn4

== system Two_Zone_MVDC_PSolver/PGM2/Subsystem ==
  Controlled Current Source : fl_lib/Electrical/Electrical Sources/Controlled Current Source
  Controlled Current Source1 : fl_lib/Electrical/Electrical Sources/Controlled Current Source
  Controlled Current Source2 : fl_lib/Electrical/Electrical Sources/Controlled Current Source
  Electrical Reference2 : fl_lib/Electrical/Electrical Elements/Electrical Reference
  Phase Splitter : ee_lib/Connectors & References/Phase Splitter
  Three Element Demux : fl_lib/Physical Signals/Nonlinear Operators/PS Three-Element Demux
      settings: InternalSimscapePortConfiguration="{\"Bottom\":[],\"Left\":[{\"id\":\"abc\",\"label\":\"abc\",\"type\":\"input\"}],\"Right\":[{\"id\":\"a\",\"label\":\"a\",\"type\":\"output\"},{\"id\":\"b\",\"label\":\"b\",\"type\":\"output\"},{\"id\":\"c\",\"label\":\"c\",\"type\":\"output\"}],\"Top\":[]}"
  ~ : PMIOPort  Side=Right
  mod : PMIOPort  Port=2  Side=Left
  connections:
  Three Element Demux/LConn1 -- mod/RConn1
  Three Element Demux/RConn1 -- Controlled Current Source/RConn1
  Three Element Demux/RConn2 -- Controlled Current Source1/RConn1
  Controlled Current Source2/RConn1 -- Three Element Demux/RConn3
  Phase Splitter/RConn3 -- Controlled Current Source2/LConn1
  ~/RConn1 -- Phase Splitter/LConn1
  Phase Splitter/RConn2 -- Controlled Current Source1/LConn1
  Phase Splitter/RConn1 -- Controlled Current Source/LConn1
  Controlled Current Source2/RConn2 -- Controlled Current Source1/RConn2 -- Controlled Current Source/RConn2 -- Electrical Reference2/LConn1

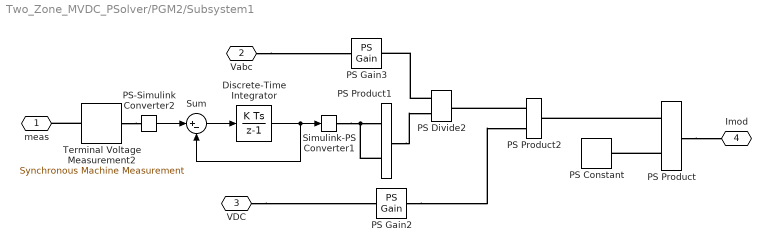
== system Two_Zone_MVDC_PSolver/PGM2/Subsystem1 ==
  Discrete-Time Integrator : DiscreteIntegrator  gainval=200  InitialCondition=1  SampleTime=-1  ICPrevOutput=DiscIntNeverNeededParam  ICPrevScaledInput=DiscIntNeverNeededParam
  PS Constant : fl_lib/Physical Signals/Sources/PS Constant  constant=-12/13.8 1/V/A
  PS Divide2 : fl_lib/Physical Signals/Functions/PS Divide
  PS Gain2 : fl_lib/Physical Signals/Functions/PS Gain  gain=1/12e3 1/V
  PS Gain3 : fl_lib/Physical Signals/Functions/PS Gain  gain=1/13.8e3
  PS Product : fl_lib/Physical Signals/Functions/PS Product
  PS Product1 : fl_lib/Physical Signals/Functions/PS Product
  PS Product2 : fl_lib/Physical Signals/Functions/PS Product
  PS-Simulink Converter2 : nesl_utility/PS-Simulink Converter  PhysicalDomain=network_engine_domain  SubClassName=ps_output  LeftPortType=input  RightPortType=output  PseudoPeriodic=off  Frequencies=[]  VectorFormat=1-D array  Unit=inherit  AffineConversion=off
  Simulink-PS Converter1 : nesl_utility/Simulink-PS Converter  PhysicalDomain=network_engine_domain  SubClassName=ps_input  LeftPortType=input  RightPortType=output  PseudoPeriodic=off  Frequencies=[]  NoiseDistribution=none  NoiseParameters=[]  Unit=1  AffineConversion=off  FilteringAndDerivatives=provide  SimscapeFilterOrder=1  InputFilterTimeConstant=0.001  UdotUserProvided=0
  Sum : Sum  Inputs=|+-
  Terminal Voltage Measurement2 : ee_lib/Electromechanical/Synchronous/Synchronous Machine Measurement  output_idx=14
      settings: LogSimulationData=on  InternalSimscapePortConfiguration="{\"Bottom\":[],\"Left\":[{\"id\":\"pu_input\",\"label\":\"pu\",\"type\":\"input\"}],\"Right\":[{\"id\":\"pu_output\",\"label\":\"o\",\"type\":\"output\"}],\"Top\":[]}"
  meas : PMIOPort  Side=Left
  Vabc : PMIOPort  Port=2  Side=Left
  VDC : PMIOPort  Port=3  Side=Right
  Imod : PMIOPort  Port=4  Side=Right
  wires:
  Sum/1 -> Discrete-Time Integrator/1
  Discrete-Time Integrator/1 -> Sum/2, Simulink-PS Converter1/1
  PS-Simulink Converter2/1 -> Sum/1
  connections:
  PS Product1/RConn1 -- PS Divide2/LConn2
  PS Product/LConn1 -- PS Product2/RConn1
  Vabc/RConn1 -- PS Gain3/LConn1
  PS Gain2/RConn1 -- PS Product2/LConn2
  PS Product/RConn1 -- Imod/RConn1
  VDC/RConn1 -- PS Gain2/LConn1
  PS Product2/LConn1 -- PS Divide2/RConn1
  PS Product/LConn2 -- PS Constant/RConn1
  Terminal Voltage Measurement2/LConn1 -- meas/RConn1
  PS Divide2/LConn1 -- PS Gain3/RConn1
  Terminal Voltage Measurement2/RConn1 -- PS-Simulink Converter2/LConn1
  Simulink-PS Converter1/RConn1 -- PS Product1/LConn2 -- PS Product1/LConn1

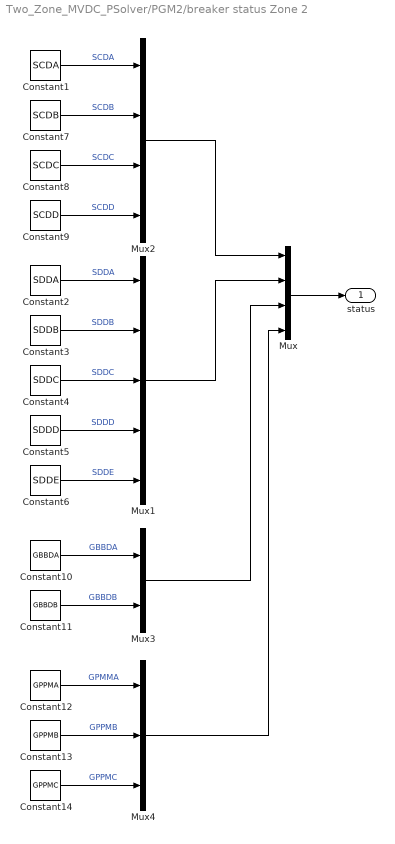
== system Two_Zone_MVDC_PSolver/PGM2/breaker status Zone 2 ==
  Constant1 : Constant  Value=SCDA  SampleTime=Ts
  Constant10 : Constant  Value=GBBDA  SampleTime=Ts
  Constant11 : Constant  Value=GBBDB  SampleTime=Ts
  Constant12 : Constant  Value=GPPMA  SampleTime=Ts
  Constant13 : Constant  Value=GPPMB  SampleTime=Ts
  Constant14 : Constant  Value=GPPMC  SampleTime=Ts
  Constant2 : Constant  Value=SDDA  SampleTime=Ts
  Constant3 : Constant  Value=SDDB  SampleTime=Ts
  Constant4 : Constant  Value=SDDC  VectorParams1D=off  SampleTime=Ts
  Constant5 : Constant  Value=SDDD  SampleTime=Ts
  Constant6 : Constant  Value=SDDE  SampleTime=Ts
  Constant7 : Constant  Value=SCDB  SampleTime=Ts
  Constant8 : Constant  Value=SCDC  SampleTime=Ts
  Constant9 : Constant  Value=SCDD  SampleTime=Ts
  Mux : Mux  Inputs=[4 5 2 3]
  Mux1 : Mux  Inputs=5
  Mux2 : Mux
  Mux3 : Mux  Inputs=2
  Mux4 : Mux  Inputs=3
  status : Outport  VectorParamsAs1DForOutWhenUnconnected=off
  wires:
  Mux/1 -> status/1
  Constant9/1 -> Mux2/4  "SCDD"
  Constant8/1 -> Mux2/3  "SCDC"
  Constant7/1 -> Mux2/2  "SCDB"
  Constant1/1 -> Mux2/1  "SCDA"
  Constant6/1 -> Mux1/5  "SDDE"
  Constant4/1 -> Mux1/3  "SDDC"
  Constant3/1 -> Mux1/2  "SDDB"
  Constant2/1 -> Mux1/1  "SDDA"
  Constant5/1 -> Mux1/4  "SDDD"
  Constant10/1 -> Mux3/1  "GBBDA"
  Constant11/1 -> Mux3/2  "GBBDB"
  Constant12/1 -> Mux4/1  "GPMMA"
  Constant13/1 -> Mux4/2  "GPPMB"
  Constant14/1 -> Mux4/3  "GPPMC"
  Mux2/1 -> Mux/1
  Mux1/1 -> Mux/2
  Mux3/1 -> Mux/3
  Mux4/1 -> Mux/4

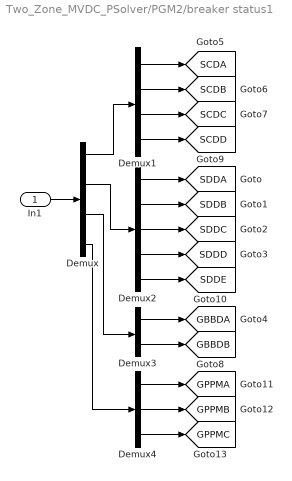
== system Two_Zone_MVDC_PSolver/PGM2/breaker status1 ==
  In1 : Inport
  Demux : Demux  Outputs=[4 5 2 3]
  Demux1 : Demux
  Demux2 : Demux  Outputs=5
  Demux3 : Demux  Outputs=2
  Demux4 : Demux  Outputs=3
  tag scope: GBBDA=global, GBBDB=global, GPPMA=global, GPPMB=global, GPPMC=global, SCDA=global, SCDB=global, SCDC=global, SCDD=global, SDDA=global, SDDB=global, SDDC=global, SDDD=global, SDDE=global
  wires:
  Demux/4 -> Demux4/1
  Demux4/3 -> [GPPMC]
  Demux4/2 -> [GPPMB]
  Demux4/1 -> [GPPMA]
  Demux/3 -> Demux3/1
  Demux3/2 -> [GBBDB]
  Demux3/1 -> [GBBDA]
  Demux/2 -> Demux2/1
  Demux/1 -> Demux1/1
  Demux2/5 -> [SDDE]
  Demux1/4 -> [SCDD]
  Demux1/3 -> [SCDC]
  Demux1/2 -> [SCDB]
  Demux1/1 -> [SCDA]
  In1/1 -> Demux/1
  Demux2/4 -> [SDDD]
  Demux2/3 -> [SDDC]
  Demux2/1 -> [SDDA]
  Demux2/2 -> [SDDB]
